simulink model "ex_1_v1"  (R2024b)
settings: Solver=FixedStepAuto  StartTime=0.0  StopTime=10.0  FixedStep=1e-3  RelTol=1e-3
undefined symbols (not defined in the file): A, B, C, D, kd, ki, kp, tl
settings Model: Creator=andre  LastModifiedBy=farin

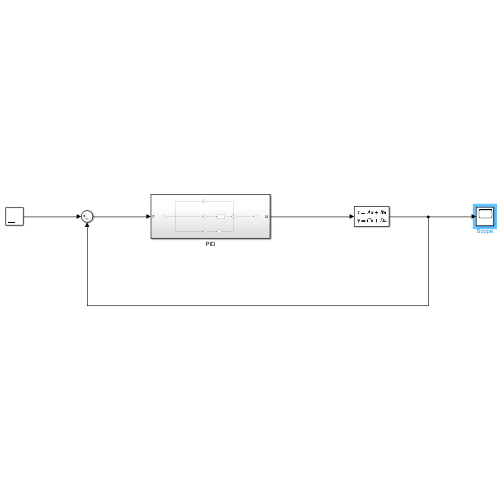
[thumbnail: Simulink's stored preview of the top-level diagram]
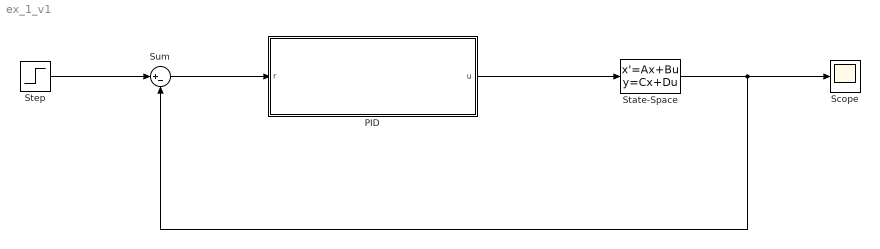
== system ex_1_v1 ==
  PID : Subsystem
  Scope : Scope
  State-Space : StateSpace  A=A  B=B  C=C  D=D  InitialCondition=0
  Step : Step  After=100  SampleTime=0
  Sum : Sum  Inputs=|+-
  wires:
  Sum/1 -> PID/1(r)
  Step/1 -> Sum/1
  State-Space/1 -> Sum/2, Scope/1
  PID/1(u) -> State-Space/1

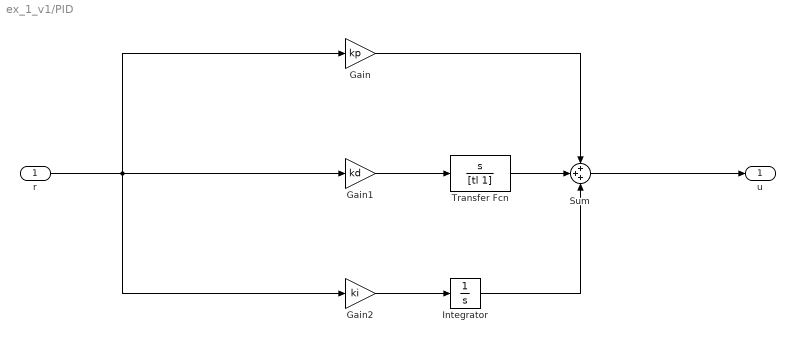
== system ex_1_v1/PID ==
  r : Inport
  Gain : Gain  Gain=kp
  Gain1 : Gain  Gain=kd
  Gain2 : Gain  Gain=ki
  Integrator : Integrator
  Sum : Sum  Inputs=+++
  Transfer Fcn : TransferFcn  Numerator=[1 0]  Denominator=[tl 1]
  u : Outport
  wires:
  Sum/1 -> u/1
  r/1 -> Gain2/1, Gain/1, Gain1/1
  Gain/1 -> Sum/1
  Transfer Fcn/1 -> Sum/2
  Integrator/1 -> Sum/3
  Gain2/1 -> Integrator/1
  Gain1/1 -> Transfer Fcn/1
